simulink model "CaseStudyII_9_Bus"  (R2020a)
settings: Solver=FixedStepAuto  StartTime=0.0  StopTime=Tend  FixedStep=T_s_power  MaxStep=5.0E-5  RelTol=1e-3
values from neighbouring files (symbols this model uses):
  B_s46 = b_s46*Cb    (= 9.5071761847e-07)    [Data_CaseStudyI.m]    (also in Data_CaseStudyII.m; Data_InitialSystem.m)
  B_s54 = b_s54*Cb    (= 1.05902722057e-06)    [Data_CaseStudyI.m]    (also in Data_CaseStudyII.m; Data_InitialSystem.m)
  B_s69 = b_s69*Cb    (= 2.15415764185e-06)    [Data_CaseStudyI.m]    (also in Data_CaseStudyII.m; Data_InitialSystem.m)
  B_s75 = b_s75*Cb    (= 1.84126323577e-06)    [Data_CaseStudyI.m]    (also in Data_CaseStudyII.m; Data_InitialSystem.m)
  B_s87 = b_s87*Cb    (= 8.96562817417e-07)    [Data_CaseStudyI.m]    (also in Data_CaseStudyII.m; Data_InitialSystem.m)
  B_s98 = b_s98*Cb    (= 1.25759482443e-06)    [Data_CaseStudyI.m]    (also in Data_CaseStudyII.m; Data_InitialSystem.m)
  C_dc_DVPP_1_2 = 0.008*(n_DVPP_1_2)    (= 0.8)    [Data_CaseStudyI.m]    (also in Data_CaseStudyII.m)
  C_dc_DVPP_1_3 = 0.008*(n_DVPP_1_3)    (= 0.4)    [Data_CaseStudyI.m]    (also in Data_CaseStudyII.m)
  C_dc_DVPP_3_1 = 0.008*(n_DVPP_3_1)    (= 1.128)    [Data_CaseStudyII.m]
  C_dc_DVPP_3_2 = 0.008*(n_DVPP_3_2)    (= 0.848)    [Data_CaseStudyII.m]
  C_dc_DVPP_3_3 = 0.008*(n_DVPP_3_3)    (= 1.28)    [Data_CaseStudyII.m]
  Dp_DVPP_3_pu = 1/dp_DVPP_3    (= 33.3333333333)    [Data_CaseStudyII.m]
  Dq1_DVPP_3_pu = 100    [Data_CaseStudyII.m]
  fb = 50    [Data_CaseStudyI.m]    (also in Data_CaseStudyII.m; Data_InitialSystem.m)
  HGov_dyn = HGov_delay*H_tr_droop    [Data_CaseStudyI.m]    (also in Data_CaseStudyII.m; Data_InitialSystem.m)
  HTurb_tot = H_water_way    [Data_CaseStudyI.m]    (also in Data_CaseStudyII.m; Data_InitialSystem.m)
  I_m_DVPP_1_2 = 2/3*Sb_DVPP_1_2/V_m_DVPP_1_2    [Data_CaseStudyI.m]    (also in Data_CaseStudyII.m)
  I_m_DVPP_1_3 = 2/3*Sb_DVPP_1_3/V_m_DVPP_1_3    [Data_CaseStudyI.m]    (also in Data_CaseStudyII.m)
  I_m_DVPP_3_1 = 2/3*Sb_DVPP_3_1/V_m_DVPP_3_1    [Data_CaseStudyII.m]
  I_m_DVPP_3_2 = 2/3*Sb_DVPP_3_2/V_m_DVPP_3_2    [Data_CaseStudyII.m]
  I_m_DVPP_3_3 = 2/3*Sb_DVPP_3_3/V_m_DVPP_3_3    [Data_CaseStudyII.m]
  i_star_max = 1.3    [Data_CaseStudyI.m]    (also in Data_CaseStudyII.m)
  iabc_DVPP_1_2_0 = T0*idq0_DVPP_1_2    [Data_CaseStudyI.m]    (also in Data_CaseStudyII.m)
  iabc_DVPP_1_3_0 = T0*idq0_DVPP_1_3    [Data_CaseStudyI.m]    (also in Data_CaseStudyII.m)
  iabc_DVPP_3_1_0 = T0*idq0_DVPP_3_1    [Data_CaseStudyII.m]
  iabc_DVPP_3_2_0 = T0*idq0_DVPP_3_2    [Data_CaseStudyII.m]
  iabc_DVPP_3_3_0 = T0*idq0_DVPP_3_3    [Data_CaseStudyII.m]
  K2_DVPP_1 = [-0.0221795494247 -1.60799665656 0.160449825826 -2.94803557381 -11.8081988371 -9.75170960256 0.00463021906909 -49.1667298155]    [ControlGains_DVPP1.mat]
  K3_DVPP_1 = [-0.0591512752956 -1.61493903379 -27.2946107927 -16.2119211358 -14.3657419818 2.05688388773 -2.27328406162 0.146700393037 -150.920793597]    [ControlGains_DVPP1.mat]
  k_dc_DVPP_1_2 = eta_DVPP_1_2/(Vdc_n_DVPP_1_2*m_p_DVPP_1_2)    [Data_CaseStudyI.m]    (also in Data_CaseStudyII.m)
  k_dc_DVPP_1_3 = eta_DVPP_1_3/(Vdc_n_DVPP_1_3*m_p_DVPP_1_3)    [Data_CaseStudyI.m]    (also in Data_CaseStudyII.m)
  k_dc_DVPP_3_1 = eta_DVPP_3_1/(Vdc_n_DVPP_3_1*m_p_DVPP_3_1)    [Data_CaseStudyII.m]
  k_dc_DVPP_3_2 = eta_DVPP_3_2/(Vdc_n_DVPP_3_2*m_p_DVPP_3_2)    [Data_CaseStudyII.m]
  k_dc_DVPP_3_3 = eta_DVPP_3_3/(Vdc_n_DVPP_3_3*m_p_DVPP_3_3)    [Data_CaseStudyII.m]
  ki_i_pu = 1.19    [Data_CaseStudyI.m]    (also in Data_CaseStudyII.m)
  ki_pll = 1700    [Data_CaseStudyI.m]    (also in Data_CaseStudyII.m)
  ki_q_pu = 0.005    [Data_CaseStudyI.m]    (also in Data_CaseStudyII.m)
  kp_i_pu = 0.73    [Data_CaseStudyI.m]    (also in Data_CaseStudyII.m)
  kp_pll = 150    [Data_CaseStudyI.m]    (also in Data_CaseStudyII.m)
  kp_q_pu = 0.05    [Data_CaseStudyI.m]    (also in Data_CaseStudyII.m)
  L1_DVPP_1_2_pu = 0.0186/m_DVPP_1_2    (= 0.000372)    [Data_CaseStudyI.m]    (also in Data_CaseStudyII.m)
  L1_DVPP_1_3_pu = 0.0186/m_DVPP_1_3    (= 0.000744)    [Data_CaseStudyI.m]    (also in Data_CaseStudyII.m)
  L1_DVPP_3_1_pu = 0.0186/m_DVPP_3_1    (= 0.000263829787234)    [Data_CaseStudyII.m]
  L1_DVPP_3_2_pu = 0.0186/m_DVPP_3_2    (= 0.000350943396226)    [Data_CaseStudyII.m]
  L1_DVPP_3_3_pu = 0.0186/m_DVPP_3_3    (= 0.0002325)    [Data_CaseStudyII.m]
  l1_MVHV1 = 0    [Data_CaseStudyI.m]    (also in Data_CaseStudyII.m; Data_InitialSystem.m)
  l1_MVHV2 = 0    [Data_CaseStudyI.m]    (also in Data_CaseStudyII.m; Data_InitialSystem.m)
  l1_MVHV3 = 0    [Data_CaseStudyI.m]    (also in Data_CaseStudyII.m; Data_InitialSystem.m)
  L2_DVPP_1_2_pu = L1_DVPP_1_2_pu    (= 0.000372)    [Data_CaseStudyI.m]    (also in Data_CaseStudyII.m)
  L2_DVPP_1_3_pu = L1_DVPP_1_3_pu    (= 0.000744)    [Data_CaseStudyI.m]    (also in Data_CaseStudyII.m)
  L2_DVPP_3_1_pu = L1_DVPP_3_1_pu    (= 0.000263829787234)    [Data_CaseStudyII.m]
  L2_DVPP_3_2_pu = L1_DVPP_3_2_pu    (= 0.000350943396226)    [Data_CaseStudyII.m]
  L2_DVPP_3_3_pu = L1_DVPP_3_3_pu    (= 0.0002325)    [Data_CaseStudyII.m]
  l2_MVHV1 = l_s14    (= 0.0576)    [Data_CaseStudyI.m]    (also in Data_CaseStudyII.m; Data_InitialSystem.m)
  l2_MVHV2 = l_s72    (= 0.0625)    [Data_CaseStudyI.m]    (also in Data_CaseStudyII.m; Data_InitialSystem.m)
  l2_MVHV3 = l_s39    (= 0.0586)    [Data_CaseStudyI.m]    (also in Data_CaseStudyII.m; Data_InitialSystem.m)
  l_f_DVPP_1_2 = L_f_DVPP_1_2*w_b/Zb_DVPP_1_2    [Data_CaseStudyI.m]    (also in Data_CaseStudyII.m)
  L_f_DVPP_1_2 = (1/(n_DVPP_1_2))*600*10^-6    (= 6e-06)    [Data_CaseStudyI.m]    (also in Data_CaseStudyII.m)
  l_f_DVPP_1_3 = L_f_DVPP_1_3*w_b/Zb_DVPP_1_3    [Data_CaseStudyI.m]    (also in Data_CaseStudyII.m)
  L_f_DVPP_1_3 = (1/(n_DVPP_1_3))*600*10^-6    (= 1.2e-05)    [Data_CaseStudyI.m]    (also in Data_CaseStudyII.m)
  l_f_DVPP_3_1 = L_f_DVPP_3_1*w_b/Zb_DVPP_3_1    [Data_CaseStudyII.m]
  L_f_DVPP_3_1 = (1/(n_DVPP_3_1))*600*10^-6    (= 4.25531914894e-06)    [Data_CaseStudyII.m]
  l_f_DVPP_3_2 = L_f_DVPP_3_2*w_b/Zb_DVPP_3_2    [Data_CaseStudyII.m]
  L_f_DVPP_3_2 = (1/(n_DVPP_3_2))*600*10^-6    (= 5.66037735849e-06)    [Data_CaseStudyII.m]
  l_f_DVPP_3_3 = L_f_DVPP_3_3*w_b/Zb_DVPP_3_3    [Data_CaseStudyII.m]
  L_f_DVPP_3_3 = (1/(n_DVPP_3_3))*600*10^-6    (= 3.75e-06)    [Data_CaseStudyII.m]
  L_s46 = l_s46*Lb    (= 0.154915055408)    [Data_CaseStudyI.m]    (also in Data_CaseStudyII.m; Data_InitialSystem.m)
  L_s54 = l_s54*Lb    (= 0.143128040323)    [Data_CaseStudyI.m]    (also in Data_CaseStudyII.m; Data_InitialSystem.m)
  L_s69 = l_s69*Lb    (= 0.286256080645)    [Data_CaseStudyI.m]    (also in Data_CaseStudyII.m; Data_InitialSystem.m)
  L_s75 = l_s75*Lb    (= 0.271101346964)    [Data_CaseStudyI.m]    (also in Data_CaseStudyII.m; Data_InitialSystem.m)
  L_s87 = l_s87*Lb    (= 0.12123786945)    [Data_CaseStudyI.m]    (also in Data_CaseStudyII.m; Data_InitialSystem.m)
  L_s98 = l_s98*Lb    (= 0.16973301723)    [Data_CaseStudyI.m]    (also in Data_CaseStudyII.m; Data_InitialSystem.m)
  LPV_K1_DVPP_3 = [0.014519129833 -1.24253756746e-17 -0.00331576987938 -1.41950397655e-17 -0.00331577010739 -1.6423216922e-19 0.0145191298795 1.47256053017e-18 1.92456501739e-17 0.00968260817745 7.5102914291e-19 0.0096826081765 ... (80 elements, 8x10)]    [ControlGains_DVPP3_LPV.mat]
  LPV_K2_DVPP_3 = [0.0299413265511 -2.72480441208e-16 -0.00563144274341 -6.63344905835e-17 -0.00563144273182 -1.08918556426e-16 0.0299413268326 -1.32404731664e-16 -4.78559537004e-17 -0.00914230292149 -8.50409089014e-21 -0.00914230292147 ... (80 elements, 8x10)]    [ControlGains_DVPP3_LPV.mat]
  LPV_K3_DVPP_3 = [-0.0173301370849 5.00398589077e-17 -0.0636125194304 3.31757376688e-17 -0.0636125164794 5.41726806116e-17 -0.017330137145 2.43427565927e-17 -0.0400570975704 -5.68753124238e-17 -0.0574012283733 2.45717741258e-17 ... (192 elements, 16x12)]    [ControlGains_DVPP3_LPV.mat]
  Mp_DVPP_3_pu = 13    [Data_CaseStudyII.m]
  P_L = pL*Sb    (= 300000000)    [Data_CaseStudyI.m]    (also in Data_CaseStudyII.m; Data_InitialSystem.m)
  p_set_bus1 = P_set_bus1/SbSG1    (= 0.731707317073)    [Data_CaseStudyI.m]    (also in Data_CaseStudyII.m; Data_InitialSystem.m)
  p_set_bus2 = P_set_bus2/SbSG2    (= 0.756707317073)    [Data_CaseStudyI.m]    (also in Data_CaseStudyII.m; Data_InitialSystem.m)
  Pb_DVPP_3_1 = 37e6    (= 37000000)    [Data_CaseStudyII.m]
  Pb_DVPP_3_2 = 28e6    (= 28000000)    [Data_CaseStudyII.m]
  Pb_DVPP_3_3 = 0e6    (= 0)    [Data_CaseStudyII.m]
  pset_DVPP_1_1 = P_set_bus1/SbSG1    (= 0.731707317073)    [Data_CaseStudyI.m]    (also in Data_CaseStudyII.m)
  pset_DVPP_1_2 = 0    [Data_CaseStudyI.m]    (also in Data_CaseStudyII.m)
  pset_DVPP_1_3 = 0    [Data_CaseStudyI.m]    (also in Data_CaseStudyII.m)
  pset_DVPP_3_1 = (0.6*P_set_bus3)/Sb_DVPP_3_1    (= 0.398546964193)    [Data_CaseStudyII.m]
  pset_DVPP_3_2 = (0.4*P_set_bus3)/Sb_DVPP_3_2    (= 0.353428439945)    [Data_CaseStudyII.m]
  pset_DVPP_3_3 = 0    [Data_CaseStudyII.m]
  Q_L = qL*Sb    (= 82500000)    [Data_CaseStudyI.m]    (also in Data_CaseStudyII.m; Data_InitialSystem.m)
  qset_DVPP_1_2 = 0    [Data_CaseStudyI.m]    (also in Data_CaseStudyII.m)
  qset_DVPP_1_3 = 0    [Data_CaseStudyI.m]    (also in Data_CaseStudyII.m)
  qset_DVPP_3_1 = 0    [Data_CaseStudyII.m]
  qset_DVPP_3_2 = 0    [Data_CaseStudyII.m]
  qset_DVPP_3_3 = 0    [Data_CaseStudyII.m]
  R1_DVPP_1_2_pu = 0.00734/m_DVPP_1_2    (= 0.0001468)    [Data_CaseStudyI.m]    (also in Data_CaseStudyII.m)
  R1_DVPP_1_3_pu = 0.00734/m_DVPP_1_3    (= 0.0002936)    [Data_CaseStudyI.m]    (also in Data_CaseStudyII.m)
  R1_DVPP_3_1_pu = 0.00734/m_DVPP_3_1    (= 0.000104113475177)    [Data_CaseStudyII.m]
  R1_DVPP_3_2_pu = 0.00734/m_DVPP_3_2    (= 0.000138490566038)    [Data_CaseStudyII.m]
  R1_DVPP_3_3_pu = 0.00734/m_DVPP_3_3    (= 9.175e-05)    [Data_CaseStudyII.m]
  r1_MVHV1 = 1e-6    (= 1e-06)    [Data_CaseStudyI.m]    (also in Data_CaseStudyII.m; Data_InitialSystem.m)
  r1_MVHV2 = 1e-6    (= 1e-06)    [Data_CaseStudyI.m]    (also in Data_CaseStudyII.m; Data_InitialSystem.m)
  r1_MVHV3 = 1e-6    (= 1e-06)    [Data_CaseStudyI.m]    (also in Data_CaseStudyII.m; Data_InitialSystem.m)
  R2_DVPP_1_2_pu = R1_DVPP_1_2_pu    (= 0.0001468)    [Data_CaseStudyI.m]    (also in Data_CaseStudyII.m)
  R2_DVPP_1_3_pu = R1_DVPP_1_3_pu    (= 0.0002936)    [Data_CaseStudyI.m]    (also in Data_CaseStudyII.m)
  R2_DVPP_3_1_pu = R1_DVPP_3_1_pu    (= 0.000104113475177)    [Data_CaseStudyII.m]
  R2_DVPP_3_2_pu = R1_DVPP_3_2_pu    (= 0.000138490566038)    [Data_CaseStudyII.m]
  R2_DVPP_3_3_pu = R1_DVPP_3_3_pu    (= 9.175e-05)    [Data_CaseStudyII.m]
  r2_MVHV1 = 1e-6    (= 1e-06)    [Data_CaseStudyI.m]    (also in Data_CaseStudyII.m; Data_InitialSystem.m)
  r2_MVHV2 = 1e-6    (= 1e-06)    [Data_CaseStudyI.m]    (also in Data_CaseStudyII.m; Data_InitialSystem.m)
  r2_MVHV3 = 1e-6    (= 1e-06)    [Data_CaseStudyI.m]    (also in Data_CaseStudyII.m; Data_InitialSystem.m)
  R_dc_DVPP_1_2 = (Vdc_n_DVPP_1_2/(0.05*(Sb_DVPP_1_2)/Vdc_n_DVPP_1_2))    [Data_CaseStudyI.m]    (also in Data_CaseStudyII.m)
  R_dc_DVPP_1_3 = (Vdc_n_DVPP_1_3/(0.05*(Sb_DVPP_1_3)/Vdc_n_DVPP_1_3))    [Data_CaseStudyI.m]    (also in Data_CaseStudyII.m)
  R_dc_DVPP_3_1 = (Vdc_n_DVPP_3_1/(0.05*(Sb_DVPP_3_1)/Vdc_n_DVPP_3_1))    [Data_CaseStudyII.m]
  R_dc_DVPP_3_2 = (Vdc_n_DVPP_3_2/(0.05*(Sb_DVPP_3_2)/Vdc_n_DVPP_3_2))    [Data_CaseStudyII.m]
  R_dc_DVPP_3_3 = (Vdc_n_DVPP_3_3/(0.05*(Sb_DVPP_3_3)/Vdc_n_DVPP_3_3))    [Data_CaseStudyII.m]
  r_f_DVPP_1_2 = R_f_DVPP_1_2/Zb_DVPP_1_2    [Data_CaseStudyI.m]    (also in Data_CaseStudyII.m)
  R_f_DVPP_1_2 = 0.02/n_DVPP_1_2    (= 0.0002)    [Data_CaseStudyI.m]    (also in Data_CaseStudyII.m)
  r_f_DVPP_1_3 = R_f_DVPP_1_3/Zb_DVPP_1_3    [Data_CaseStudyI.m]    (also in Data_CaseStudyII.m)
  R_f_DVPP_1_3 = 0.02/n_DVPP_1_3    (= 0.0004)    [Data_CaseStudyI.m]    (also in Data_CaseStudyII.m)
  r_f_DVPP_3_1 = R_f_DVPP_3_1/Zb_DVPP_3_1    [Data_CaseStudyII.m]
  ... (+104 more)
undefined symbols (not defined in the file or in its folder): A, B, C, Continuous, Dd, Efd0, gcbh, i_dc, Ka, Kf, p2set, SbSM2, sps_rtmsupport, spsST1AModel, Ta, Tb, Tb1, Tc, Tc1, Tf, VA0, VAmax, VAmin, VImax, VImin, VRmax, VRmin
libraries: powerlib x95, powerlib_meascontrol x41, cstblocks x15, sps_avr x1, simulink_extras x1, simulink x1
(part 4 of 5)

== system CaseStudyII_9_Bus/STATCOM with Battery/Power Controllers1 ==
  Q_abc : Inport
  Delta x_c : Inport  Port=2
  w_pll : Inport  Port=3
  P_abc : Inport  Port=4
  P_set : Inport  Port=5
  |V| : Inport  Port=6
  Q_set : Inport  Port=7
  theta1_p : Inport  Port=8
  theta2_p : Inport  Port=9
  theta3_q : Inport  Port=10
  0 : Constant  Value=0
  DVPP State Feedback Controller : Subsystem
  Mux : Mux  Inputs=3
  i_star_dq0 : Outport
  p_des : Outport  Port=2
  q_des : Outport  Port=3
  PQ_des_DVPP3 : Outport  Port=4
  wires:
  0/1 -> Mux/3
  DVPP State Feedback Controller/1(i_star_d) -> Mux/1
  DVPP State Feedback Controller/3(p_des) -> p_des/1
  Q_abc/1 -> DVPP State Feedback Controller/5(Q_abc)
  |V|/1 -> DVPP State Feedback Controller/2("|V| ")
  DVPP State Feedback Controller/2(i_star_q) -> Mux/2
  DVPP State Feedback Controller/4(q_des) -> q_des/1
  w_pll/1 -> DVPP State Feedback Controller/1(w_pll)
  P_abc/1 -> DVPP State Feedback Controller/3(P_abc)
  P_set/1 -> DVPP State Feedback Controller/4(P_set)
  Delta x_c/1 -> DVPP State Feedback Controller/6(Delta_x_c)
  Mux/1 -> i_star_dq0/1
  Q_set/1 -> DVPP State Feedback Controller/7(Q_set)
  theta1_p/1 -> DVPP State Feedback Controller/8(theta1_p)
  theta2_p/1 -> DVPP State Feedback Controller/9(theta2_q)
  theta3_q/1 -> DVPP State Feedback Controller/10(theta3_q)
  DVPP State Feedback Controller/5(PQ_des_DVPP3) -> PQ_des_DVPP3/1

== system CaseStudyII_9_Bus/STATCOM with Battery/Reference current limitation ==
  i_star_dq0 : Inport
  i_star_max : Inport  Port=2
  Demux1 : Demux  Outputs=3
  Demux2 : Demux  Outputs=3
  Divide : Product  Inputs=*/
  Minus : Sum  Inputs=+-
  Minus1 : Sum  Inputs=+++
  Minus4 : Sum  Inputs=+++
  Product{,1..4,6..7} (7 alike) : Product  RndMeth=Zero
  Saturation1 : Saturate  UpperLimit=inf  LowerLimit=0
  Sign : Signum
  Sqrt1 : Sqrt  SaturateOnIntegerOverflow=on
  Sqrt2 : Sqrt  SaturateOnIntegerOverflow=on
  Switch1 : Switch  Threshold=1
  i_star_dq0_lim : Outport  VectorParamsAs1DForOutWhenUnconnected=off
  ||i_star_dq0|| : Outport  Port=2  VectorParamsAs1DForOutWhenUnconnected=off
  ||i_star_dq0_lim|| : Outport  Port=3  VectorParamsAs1DForOutWhenUnconnected=off
  wires:
  Sqrt2/1 -> ||i_star_dq0_lim||/1
  Minus1/1 -> Sqrt2/1
  Demux2/2 -> Product3/2, Product3/1
  Product3/1 -> Minus1/2
  Demux2/1 -> Product2/1, Product2/2
  Product4/1 -> Minus1/3
  Demux2/3 -> Product4/2, Product4/1
  Product2/1 -> Minus1/1
  i_star_max/1 -> Product6/2, Minus/2
  i_star_dq0/1 -> Switch1/3, Demux1/1, Divide/1
  Demux1/3 -> Product7/2, Product7/1
  Product7/1 -> Minus4/3
  Product6/1 -> Switch1/1
  Divide/1 -> Product6/1
  Sign/1 -> Switch1/2
  Saturation1/1 -> Sign/1
  Demux1/2 -> Product1/2, Product1/1
  Product/1 -> Minus4/1
  Product1/1 -> Minus4/2
  Demux1/1 -> Product/1, Product/2
  Minus4/1 -> Sqrt1/1
  Sqrt1/1 -> Minus/1, ||i_star_dq0||/1, Divide/2
  Minus/1 -> Saturation1/1
  Switch1/1 -> Demux2/1, i_star_dq0_lim/1

== system CaseStudyII_9_Bus/Supercapacitor/Converter State Deviation ==
  i_dq0 : Inport
  x_id : Inport  Port=2
  pset : Inport  Port=3
  Constant1 : Constant  Value=xid0_DVPP_1_3_pu
  Demux2 : Demux  Outputs=3
  Gain : Gain  Gain=1/vd0_DVPP_1_3_pu
  Mux : Mux  Inputs=2
  Sum : Sum  Inputs=-+|
  Sum1 : Sum  Inputs=|+-
  Delta x_c : Outport
  wires:
  i_dq0/1 -> Demux2/1
  pset/1 -> Gain/1
  Sum/1 -> Mux/1
  Demux2/1 -> Sum/2
  Gain/1 -> Sum/1
  x_id/1 -> Sum1/1
  Constant1/1 -> Sum1/2
  Mux/1 -> Delta x_c/1
  Sum1/1 -> Mux/2

== system CaseStudyII_9_Bus/Supercapacitor/Current Loop ==
  i_star_dq0 : Inport
  v_dq0 : Inport  Port=2
  i_dq0 : Inport  Port=3
  w_pll : Inport  Port=4
  Demux : Demux  Outputs=2
  Demux1 : Demux  Outputs=2
  Demux2 : Demux  Outputs=2
  Gain : Gain  Gain=kp_i_pu
  Gain1 : Gain  Gain=ki_i_pu
  Gain2 : Gain  Gain=kp_i_pu
  Gain3 : Gain  Gain=ki_i_pu
  Gain4 : Gain  Gain=w_b
  Integrator1 : Integrator  InitialCondition=xid0_DVPP_1_3_pu
  Integrator2 : Integrator  InitialCondition=xiq0_DVPP_1_3_pu
  Memory2 : Memory
  Mux : Mux  Inputs=3
  Product : Product
  Product1 : Product
  Rf : Gain  Gain=r_f_DVPP_1_3
  Rf1 : Gain  Gain=r_f_DVPP_1_3
  Selector1 : Selector  InputPortWidth=3  IndexOptions=Index vector (dialog)  Indices=[1 2]  OutputSizes=1
  Selector2 : Selector  InputPortWidth=3  IndexOptions=Index vector (dialog)  Indices=[1 2]  OutputSizes=1
  Selector3 : Selector  InputPortWidth=3  IndexOptions=Index vector (dialog)  Indices=[1 2]  OutputSizes=1
  Sum : Sum  Inputs=|+-
  Sum1 : Sum
  Sum2 : Sum  Inputs=|+-+
  Sum3 : Sum  Inputs=|++
  Sum4 : Sum
  Sum5 : Sum  Inputs=+++|
  Sum6 : Sum  Inputs=-+|
  Sum7 : Sum  Inputs=++|
  vs_0* : Constant  Value=0
  w*Lf : Gain  Gain=l_f_DVPP_1_3/w_b
  w*Lf1 : Gain  Gain=l_f_DVPP_1_3/w_b
  v_s_ref_dq0 : Outport  VectorParamsAs1DForOutWhenUnconnected=off
  x_id : Outport  Port=2  VectorParamsAs1DForOutWhenUnconnected=off
  wires:
  vs_0*/1 -> Mux/3
  Selector3/1 -> Demux2/1
  i_dq0/1 -> Selector2/1
  Selector2/1 -> Demux1/1
  Mux/1 -> v_s_ref_dq0/1
  Sum2/1 -> Sum3/1
  v_dq0/1 -> Selector3/1
  i_star_dq0/1 -> Selector1/1
  w*Lf/1 -> Sum2/2
  Sum7/1 -> Mux/2  "vs_q*"
  Sum3/1 -> Mux/1  "vs_d*"
  Sum5/1 -> Sum7/2
  Rf/1 -> Sum2/3
  Rf1/1 -> Sum5/3
  Sum/1 -> Integrator1/1, Gain/1
  Sum1/1 -> Sum2/1
  Selector1/1 -> Demux/1
  Demux/2 -> Sum6/2
  Demux/1 -> Sum/1
  w*Lf1/1 -> Sum5/1
  Demux2/1 -> Sum3/2
  Demux2/2 -> Sum7/1
  Demux1/1 -> Product/1, Rf/1, Sum/2
  Demux1/2 -> Product1/1, Rf1/1, Sum6/1
  Gain/1 -> Sum1/1
  Gain1/1 -> Sum1/2
  Gain2/1 -> Sum4/1
  Sum6/1 -> Integrator2/1, Gain2/1
  Sum4/1 -> Sum5/2
  Gain3/1 -> Sum4/2
  Integrator2/1 -> Gain3/1
  Integrator1/1 -> Memory2/1, Gain1/1
  w_pll/1 -> Gain4/1
  Product/1 -> w*Lf1/1
  Product1/1 -> w*Lf/1
  Gain4/1 -> Product1/2, Product/2
  Memory2/1 -> x_id/1

== system CaseStudyII_9_Bus/Supercapacitor/PLL ==
  v_abc : Inport
  Display : Display
  Gain : Gain  Gain=1/fb
  Integrator3 : Integrator  InitialCondition=xpll0_pu
  Selector : Selector  InputPortWidth=3  IndexOptions=Index vector (dialog)  Indices=2  OutputSizes=1
  Subsystem : Subsystem
  abc to dq0 : powerlib_meascontrol/Transformations/abc to dq0  Alignment=90 degrees behind phase A axis
  theta_pll : Outport  VectorParamsAs1DForOutWhenUnconnected=off
  v_dq0 : Outport  Port=2  VectorParamsAs1DForOutWhenUnconnected=off
  w_pll : Outport  Port=3  VectorParamsAs1DForOutWhenUnconnected=off
  x_pll : Outport  Port=4  VectorParamsAs1DForOutWhenUnconnected=off
  wires:
  Gain/1 -> w_pll/1
  Integrator3/1 -> x_pll/1
  v_abc/1 -> Subsystem/1(Vabc), abc to dq0/1
  abc to dq0/1 -> Selector/1, v_dq0/1
  Subsystem/1(Freq) -> Display/1, Gain/1
  Subsystem/2(wt) -> abc to dq0/2, theta_pll/1
  Selector/1 -> Integrator3/1

== system CaseStudyII_9_Bus/Supercapacitor/Power Controllers ==
  Q_abc : Inport
  w_pll : Inport  Port=2
  P_abc : Inport  Port=3
  Q_set : Inport  Port=4
  Delta x_c : Inport  Port=5
  P_set : Inport  Port=6
  0 : Constant  Value=0
  DVPP State Feedback Controller for Active Power Control : Subsystem
  Mux : Mux  Inputs=3
  Reactive Power Controller PI-droop control : Subsystem
  i_star_dq0 : Outport
  p_des : Outport  Port=2
  wires:
  Mux/1 -> i_star_dq0/1
  0/1 -> Mux/3
  DVPP State Feedback Controller for Active Power Control/2(i_star_d) -> Mux/1
  DVPP State Feedback Controller for Active Power Control/1(p_des) -> p_des/1
  w_pll/1 -> DVPP State Feedback Controller for Active Power Control/1(w_pll)
  P_abc/1 -> DVPP State Feedback Controller for Active Power Control/2(P_abc)
  Reactive Power Controller PI-droop control/1(i_star_q) -> Mux/2
  Q_abc/1 -> Reactive Power Controller PI-droop control/1(Q_abc)
  Q_set/1 -> Reactive Power Controller PI-droop control/2(Qset)
  Delta x_c/1 -> DVPP State Feedback Controller for Active Power Control/3(Delta_x_c)
  P_set/1 -> DVPP State Feedback Controller for Active Power Control/4(P_set)

== system CaseStudyII_9_Bus/Supercapacitor/Reference current limitation ==
  i_star_dq0 : Inport
  i_star_max : Inport  Port=2
  Demux1 : Demux  Outputs=3
  Demux2 : Demux  Outputs=3
  Divide : Product  Inputs=*/
  Minus : Sum  Inputs=+-
  Minus1 : Sum  Inputs=+++
  Minus4 : Sum  Inputs=+++
  Product{,1..4,6..7} (7 alike) : Product  RndMeth=Zero
  Saturation1 : Saturate  UpperLimit=inf  LowerLimit=0
  Sign : Signum
  Sqrt1 : Sqrt  SaturateOnIntegerOverflow=on
  Sqrt2 : Sqrt  SaturateOnIntegerOverflow=on
  Switch1 : Switch  Threshold=1
  i_star_dq0_lim : Outport  VectorParamsAs1DForOutWhenUnconnected=off
  ||i_star_dq0|| : Outport  Port=2  VectorParamsAs1DForOutWhenUnconnected=off
  ||i_star_dq0_lim|| : Outport  Port=3  VectorParamsAs1DForOutWhenUnconnected=off
  wires:
  Sqrt2/1 -> ||i_star_dq0_lim||/1
  Minus1/1 -> Sqrt2/1
  Demux2/2 -> Product3/2, Product3/1
  Product3/1 -> Minus1/2
  Demux2/1 -> Product2/1, Product2/2
  Product4/1 -> Minus1/3
  Demux2/3 -> Product4/2, Product4/1
  Product2/1 -> Minus1/1
  i_star_max/1 -> Product6/2, Minus/2
  i_star_dq0/1 -> Switch1/3, Demux1/1, Divide/1
  Switch1/1 -> i_star_dq0_lim/1, Demux2/1
  Demux1/3 -> Product7/2, Product7/1
  Product7/1 -> Minus4/3
  Product6/1 -> Switch1/1
  Divide/1 -> Product6/1
  Sign/1 -> Switch1/2
  Saturation1/1 -> Sign/1
  Demux1/2 -> Product1/2, Product1/1
  Product/1 -> Minus4/1
  Product1/1 -> Minus4/2
  Demux1/1 -> Product/1, Product/2
  Minus4/1 -> Sqrt1/1
  Sqrt1/1 -> Minus/1, ||i_star_dq0||/1, Divide/2
  Minus/1 -> Saturation1/1

== system CaseStudyII_9_Bus/Synchronous Generator 1 Hydro Turbine/Govenor ==
  speed_ref : Inport
  speed : Inport  Port=2
  P_set : Inport  Port=3
  1/droop : Gain  Gain=(-1/Rg)
  Delta speed : Sum  Inputs=-+|
  Govenor Dynamics : cstblocks/LTI System  sys=ss(HGov_dyn)  IC=[1 1.0617]
  Sum : Sum  Inputs=++|
  throttle : Outport  VectorParamsAs1DForOutWhenUnconnected=off
  wires:
  speed/1 -> Delta speed/2
  speed_ref/1 -> Delta speed/1
  Govenor Dynamics/1 -> throttle/1
  Delta speed/1 -> 1/droop/1
  Sum/1 -> Govenor Dynamics/1
  1/droop/1 -> Sum/2  "Pm"
  P_set/1 -> Sum/1

== system CaseStudyII_9_Bus/Synchronous Machine 2 reheat steam turbine/Govenor ==
  speed_ref : Inport
  speed : Inport  Port=2
  P_set : Inport  Port=3
  1/droop : Gain  Gain=(-1/Rg)
  Delta speed : Sum  Inputs=-+|
  Govenor Dynamics : cstblocks/LTI System  sys=ss(SGov_dyn)  IC=[p_set_bus2/2.5]
  Sum : Sum  Inputs=++|
  throttle : Outport  VectorParamsAs1DForOutWhenUnconnected=off
  wires:
  speed/1 -> Delta speed/2
  speed_ref/1 -> Delta speed/1
  Govenor Dynamics/1 -> throttle/1
  Delta speed/1 -> 1/droop/1
  1/droop/1 -> Sum/2  "Pm"
  Sum/1 -> Govenor Dynamics/1
  P_set/1 -> Sum/1

== system CaseStudyII_9_Bus/Synchronous Machine 2 reheat steam turbine/ST1A Excitation System ==
  Vref : Inport
  Vt : Inport  Port=2
  Ifd : Inport  Port=3
  Vstab : Inport  Port=4
  Model : Subsystem  AncestorBlock=spsST1AModel/Continuous  mask(Excitation System){}
  Efd : Outport  VectorParamsAs1DForOutWhenUnconnected=off
  wires:
  Vstab/1 -> Model/4(Vstab)
  Ifd/1 -> Model/3(Ifd)
  Vref/1 -> Model/1(Vref)
  Vt/1 -> Model/2(Vt)
  Model/1(Efd) -> Efd/1

== system CaseStudyII_9_Bus/Wind /Converter State Deviation for DVPP with DC side1 ==
  i_dq0 : Inport
  Pset : Inport  Port=2
  Qset : Inport  Port=3
  x_id : Inport  Port=4
  x_iq : Inport  Port=5
  Demux2 : Demux  Outputs=3
  Gain : Gain  Gain=1/vd0_DVPP_3_1_pu
  Gain1 : Gain  Gain=-1/vd0_DVPP_3_1_pu
  Mux : Mux
  Sum1 : Sum  Inputs=+-
  Sum2 : Sum  Inputs=-+
  Sum3 : Sum  Inputs=+-
  Sum4 : Sum  Inputs=+-
  x_id_1_pu : Constant  Value=xid0_DVPP_3_1_pu
  x_iq_1_pu : Constant  Value=xiq0_DVPP_3_1_pu
  Delta x_c : Outport
  wires:
  i_dq0/1 -> Demux2/1
  Demux2/1 -> Sum2/2
  Demux2/2 -> Sum1/1
  Sum2/1 -> Mux/1
  Sum1/1 -> Mux/2
  Gain1/1 -> Sum1/2
  Pset/1 -> Gain/1
  Gain/1 -> Sum2/1
  Qset/1 -> Gain1/1
  x_id/1 -> Sum3/1
  Sum3/1 -> Mux/3
  x_id_1_pu/1 -> Sum3/2
  Mux/1 -> Delta x_c/1
  Sum4/1 -> Mux/4
  x_iq_1_pu/1 -> Sum4/2
  x_iq/1 -> Sum4/1

== system CaseStudyII_9_Bus/Wind /Current Loop ==
  i_star_dq0 : Inport
  v_dq0 : Inport  Port=2
  i_dq0 : Inport  Port=3
  w_pll : Inport  Port=4
  Demux : Demux  Outputs=2
  Demux1 : Demux  Outputs=2
  Demux2 : Demux  Outputs=2
  Gain : Gain  Gain=kp_i_pu
  Gain1 : Gain  Gain=ki_i_pu
  Gain2 : Gain  Gain=kp_i_pu
  Gain3 : Gain  Gain=ki_i_pu
  Gain4 : Gain  Gain=w_b
  Integrator1 : Integrator  InitialCondition=xid0_DVPP_3_1_pu
  Integrator2 : Integrator  InitialCondition=xiq0_DVPP_3_1_pu
  Memory1 : Memory
  Memory2 : Memory
  Mux : Mux  Inputs=3
  Product : Product
  Product1 : Product
  Rf : Gain  Gain=r_f_DVPP_3_1
  Rf1 : Gain  Gain=r_f_DVPP_3_1
  Selector1 : Selector  InputPortWidth=3  IndexOptions=Index vector (dialog)  Indices=[1 2]  OutputSizes=1
  Selector2 : Selector  InputPortWidth=3  IndexOptions=Index vector (dialog)  Indices=[1 2]  OutputSizes=1
  Selector3 : Selector  InputPortWidth=3  IndexOptions=Index vector (dialog)  Indices=[1 2]  OutputSizes=1
  Sum : Sum  Inputs=|+-
  Sum1 : Sum
  Sum2 : Sum  Inputs=|+-+
  Sum3 : Sum  Inputs=|++
  Sum4 : Sum
  Sum5 : Sum  Inputs=+++|
  Sum6 : Sum  Inputs=-+|
  Sum7 : Sum  Inputs=++|
  vs_0* : Constant  Value=0
  w*Lf : Gain  Gain=l_f_DVPP_3_1/w_b
  w*Lf1 : Gain  Gain=l_f_DVPP_3_1/w_b
  v_s_ref_dq0 : Outport  VectorParamsAs1DForOutWhenUnconnected=off
  x_id : Outport  Port=2  VectorParamsAs1DForOutWhenUnconnected=off
  x_iq : Outport  Port=3  VectorParamsAs1DForOutWhenUnconnected=off
  wires:
  vs_0*/1 -> Mux/3
  Selector3/1 -> Demux2/1
  i_dq0/1 -> Selector2/1
  Selector2/1 -> Demux1/1
  Mux/1 -> v_s_ref_dq0/1
  Sum2/1 -> Sum3/1
  v_dq0/1 -> Selector3/1
  i_star_dq0/1 -> Selector1/1
  w*Lf/1 -> Sum2/2
  Sum7/1 -> Mux/2  "vs_q*"
  Sum3/1 -> Mux/1  "vs_d*"
  Sum5/1 -> Sum7/2
  Rf/1 -> Sum2/3
  Rf1/1 -> Sum5/3
  Sum/1 -> Integrator1/1, Gain/1
  Sum1/1 -> Sum2/1
  Selector1/1 -> Demux/1
  Demux/2 -> Sum6/2
  Demux/1 -> Sum/1
  w*Lf1/1 -> Sum5/1
  Demux2/1 -> Sum3/2
  Demux2/2 -> Sum7/1
  Demux1/1 -> Product/1, Rf/1, Sum/2
  Demux1/2 -> Product1/1, Rf1/1, Sum6/1
  Gain/1 -> Sum1/1
  Gain1/1 -> Sum1/2
  Gain2/1 -> Sum4/1
  Sum6/1 -> Integrator2/1, Gain2/1
  Sum4/1 -> Sum5/2
  Gain3/1 -> Sum4/2
  Integrator2/1 -> Memory1/1, Gain3/1
  Integrator1/1 -> Memory2/1, Gain1/1
  w_pll/1 -> Gain4/1
  Product/1 -> w*Lf1/1
  Product1/1 -> w*Lf/1
  Gain4/1 -> Product1/2, Product/2
  Memory2/1 -> x_id/1
  Memory1/1 -> x_iq/1

== system CaseStudyII_9_Bus/Wind /PLL ==
  v_abc : Inport
  Display : Display
  Gain : Gain  Gain=1/fb
  Integrator3 : Integrator  InitialCondition=xpll0_pu
  Selector : Selector  InputPortWidth=3  IndexOptions=Index vector (dialog)  Indices=2  OutputSizes=1
  Subsystem : Subsystem
  abc to dq0 : powerlib_meascontrol/Transformations/abc to dq0  Alignment=90 degrees behind phase A axis
  theta_pll : Outport  VectorParamsAs1DForOutWhenUnconnected=off
  v_dq0 : Outport  Port=2  VectorParamsAs1DForOutWhenUnconnected=off
  w_pll : Outport  Port=3  VectorParamsAs1DForOutWhenUnconnected=off
  x_pll : Outport  Port=4  VectorParamsAs1DForOutWhenUnconnected=off
  wires:
  Gain/1 -> w_pll/1
  Integrator3/1 -> x_pll/1
  v_abc/1 -> Subsystem/1(Vabc), abc to dq0/1
  abc to dq0/1 -> Selector/1, v_dq0/1
  Subsystem/1(Freq) -> Display/1, Gain/1
  Subsystem/2(wt) -> abc to dq0/2, theta_pll/1
  Selector/1 -> Integrator3/1

== system CaseStudyII_9_Bus/Wind /Power Controllers1 ==
  Q_abc : Inport
  Delta x_c : Inport  Port=2
  w_pll : Inport  Port=3
  P_abc : Inport  Port=4
  P_set : Inport  Port=5
  |V| : Inport  Port=6
  Q_set : Inport  Port=7
  theta1_p : Inport  Port=8
  theta1_q : Inport  Port=9
  0 : Constant  Value=0
  DVPP State Feedback Controller : Subsystem
  Mux : Mux  Inputs=3
  i_star_dq0 : Outport
  p_des : Outport  Port=2
  q_des : Outport  Port=3
  wires:
  0/1 -> Mux/3
  DVPP State Feedback Controller/1(i_star_d) -> Mux/1
  DVPP State Feedback Controller/3(p_des) -> p_des/1
  Q_abc/1 -> DVPP State Feedback Controller/5(Q_abc)
  |V|/1 -> DVPP State Feedback Controller/2("|V| ")
  DVPP State Feedback Controller/2(i_star_q) -> Mux/2
  DVPP State Feedback Controller/4(q_des) -> q_des/1
  w_pll/1 -> DVPP State Feedback Controller/1(w_pll)
  P_abc/1 -> DVPP State Feedback Controller/3(P_abc)
  P_set/1 -> DVPP State Feedback Controller/4(P_set)
  Delta x_c/1 -> DVPP State Feedback Controller/6(Delta_x_c)
  Mux/1 -> i_star_dq0/1
  Q_set/1 -> DVPP State Feedback Controller/7(Q_set)
  theta1_q/1 -> DVPP State Feedback Controller/9(theta1_q)
  theta1_p/1 -> DVPP State Feedback Controller/8(theta1_p)

== system CaseStudyII_9_Bus/Wind /Reference current limitation ==
  i_star_dq0 : Inport
  i_star_max : Inport  Port=2
  Demux1 : Demux  Outputs=3
  Demux2 : Demux  Outputs=3
  Divide : Product  Inputs=*/
  Minus : Sum  Inputs=+-
  Minus1 : Sum  Inputs=+++
  Minus4 : Sum  Inputs=+++
  Product{,1..4,6..7} (7 alike) : Product  RndMeth=Zero
  Saturation1 : Saturate  UpperLimit=inf  LowerLimit=0
  Sign : Signum
  Sqrt1 : Sqrt  SaturateOnIntegerOverflow=on
  Sqrt2 : Sqrt  SaturateOnIntegerOverflow=on
  Switch1 : Switch  Threshold=1
  i_star_dq0_lim : Outport  VectorParamsAs1DForOutWhenUnconnected=off
  ||i_star_dq0|| : Outport  Port=2  VectorParamsAs1DForOutWhenUnconnected=off
  ||i_star_dq0_lim|| : Outport  Port=3  VectorParamsAs1DForOutWhenUnconnected=off
  wires:
  Sqrt2/1 -> ||i_star_dq0_lim||/1
  Minus1/1 -> Sqrt2/1
  Demux2/2 -> Product3/2, Product3/1
  Product3/1 -> Minus1/2
  Demux2/1 -> Product2/1, Product2/2
  Product4/1 -> Minus1/3
  Demux2/3 -> Product4/2, Product4/1
  Product2/1 -> Minus1/1
  i_star_max/1 -> Product6/2, Minus/2
  i_star_dq0/1 -> Switch1/3, Demux1/1, Divide/1
  Demux1/3 -> Product7/2, Product7/1
  Product7/1 -> Minus4/3
  Product6/1 -> Switch1/1
  Divide/1 -> Product6/1
  Sign/1 -> Switch1/2
  Saturation1/1 -> Sign/1
  Demux1/2 -> Product1/2, Product1/1
  Product/1 -> Minus4/1
  Product1/1 -> Minus4/2
  Demux1/1 -> Product/1, Product/2
  Minus4/1 -> Sqrt1/1
  Sqrt1/1 -> Minus/1, ||i_star_dq0||/1, Divide/2
  Minus/1 -> Saturation1/1
  Switch1/1 -> Demux2/1, i_star_dq0_lim/1

== system CaseStudyII_9_Bus/BESS/PLL/Subsystem ==
  Vabc : Inport  PortDimensions=3
  Constant : Constant  Value=2*pi*50
  Demux2 : Demux  Outputs=3
  Divide : Product  Inputs=/*
  First-Order Filter : powerlib_meascontrol/Filters/First-Order Filter  FilterType=Lowpass  Tc=0.081  Ts=0  Initialize=on  Vac_Init=[0, 0, fb]  Vdc_Init=0  PlotResponse=off  FreqRange="[0,  200,  1]"
  Gain : Gain  Gain=kp_pll
  Gain1 : Gain  Gain=ki_pll
  Gain10 : Gain  Gain=1/2/pi  SaturateOnIntegerOverflow=on  OutDataTypeStr=Inherit: Same as input  ParamDataTypeStr=Inherit: Same as input
  Integrator : Integrator
  Integrator1 : Integrator  InitialCondition=xpll0_pu
  Memory : Memory  InitialCondition=fb
  Selector : Selector  InputPortWidth=3  IndexOptions=Index vector (dialog)  Indices=2  OutputSizes=1
  Sqrt2 : Sqrt  SaturateOnIntegerOverflow=on
  Sum : Sum
  Sum1 : Sum  Inputs=++|
  Sum2 : Sum  Inputs=+++  InputSameDT=on  SaturateOnIntegerOverflow=on  OutDataTypeStr=Inherit: Same as first input
  abc to dq0 : powerlib_meascontrol/Transformations/abc to dq0  Alignment=90 degrees behind phase A axis
      settings: SourceProductBaseCode=MT,PS
  d²2 : Product  InputSameDT=on  RndMeth=Zero  SaturateOnIntegerOverflow=on  OutDataTypeStr=Inherit: Same as first input
  q²4 : Product  InputSameDT=on  RndMeth=Zero  SaturateOnIntegerOverflow=on  OutDataTypeStr=Inherit: Same as first input
  q²5 : Product  InputSameDT=on  RndMeth=Zero  SaturateOnIntegerOverflow=on  OutDataTypeStr=Inherit: Same as first input
  Freq : Outport  VectorParamsAs1DForOutWhenUnconnected=off
  wt : Outport  Port=2  VectorParamsAs1DForOutWhenUnconnected=off
  wires:
  Vabc/1 -> abc to dq0/1
  Integrator/1 -> wt/1, abc to dq0/2
  Memory/1 -> Freq/1
  Gain/1 -> Sum/1
  Gain1/1 -> Sum/2
  Integrator1/1 -> Gain1/1
  Demux2/1 -> d²2/1, d²2/2  "d"
  d²2/1 -> Sum2/1
  Demux2/3 -> q²5/1, q²5/2  "0"
  Demux2/2 -> q²4/1, q²4/2  "q"
  Sqrt2/1 -> Divide/1
  Sum2/1 -> Sqrt2/1
  q²5/1 -> Sum2/3
  abc to dq0/1 -> Demux2/1, Selector/1
  q²4/1 -> Sum2/2
  Selector/1 -> Divide/2  "Vq"
  Divide/1 -> Integrator1/1, Gain/1
  Gain10/1 -> First-Order Filter/1
  First-Order Filter/1 -> Memory/1
  Sum/1 -> Sum1/2  "W"
  Sum1/1 -> Integrator/1, Gain10/1  "W"
  Constant/1 -> Sum1/1

== system CaseStudyII_9_Bus/BESS/Power Controllers/DVPP State Feedback Controller for Active Power Control ==
  P_abc : Inport
  Delta_x_c : Inport  Port=2
  w_pll : Inport  Port=3
  Pset : Inport  Port=4
  Constant : Constant  Value=ReferenceSS2_DVPP_1.A  VectorParams1D=off
  Constant1 : Constant  Value=ReferenceSS2_DVPP_1.B  VectorParams1D=off
  Constant2 : Constant  Value=ReferenceSS2_DVPP_1.C  VectorParams1D=off
  Constant3 : Constant  Value=ReferenceSS2_DVPP_1.D  VectorParams1D=off
  Gain : Gain  Gain=K2_DVPP_1  Multiplication=Matrix(K*u)
  Gain1 : Gain  Gain=1/vd0_DVPP_1_2_pu
  Integrator : Integrator
  Mux : Mux  Inputs=3
  Scope : Scope
  Sum : Sum  Inputs=+-
  Sum1 : Sum  Inputs=++|
  Sum2 : Sum
  Sum3 : Sum  Inputs=-+
  Varying State Space : cstblocks/Linear Parameter Varying/Varying State Space  x0=0  xNames=''  OutputX=on  OutputDX=on
  w* [SI] : Constant
  p_des : Outport
  i_star_d : Outport  Port=2
  wires:
  Mux/1 -> Gain/1
  Varying State Space/1 -> Scope/1, Sum1/2
  Sum3/1 -> Integrator/1
  w* [SI]/1 -> Sum/2
  P_abc/1 -> Sum3/2
  Integrator/1 -> Mux/3
  Varying State Space/2 -> Mux/2
  Delta_x_c/1 -> Mux/1
  w_pll/1 -> Sum/1
  Constant/1 -> Varying State Space/2
  Constant1/1 -> Varying State Space/3
  Constant2/1 -> Varying State Space/4
  Constant3/1 -> Varying State Space/5
  Sum/1 -> Varying State Space/1
  Pset/1 -> Gain1/1, Sum1/1
  Sum1/1 -> Sum3/1, p_des/1
  Sum2/1 -> i_star_d/1
  Gain/1 -> Sum2/1
  Gain1/1 -> Sum2/2

== system CaseStudyII_9_Bus/BESS/Power Controllers/Reactive Power Controller PI-droop control ==
  Q_abc : Inport
  Qset : Inport  Port=2
  Gain : Gain  Gain=kp_q_pu
  Gain1 : Gain  Gain=ki_q_pu
  Integrator1 : Integrator  InitialCondition=xq0_DVPP_1_2_pu
  Sum : Sum  Inputs=-+
  Sum1 : Sum
  i_star_q : Outport
  wires:
  Q_abc/1 -> Sum/2
  Qset/1 -> Sum/1
  Sum/1 -> Integrator1/1, Gain/1
  Gain/1 -> Sum1/1
  Gain1/1 -> Sum1/2
  Integrator1/1 -> Gain1/1
  Sum1/1 -> i_star_q/1

== system CaseStudyII_9_Bus/PV/PLL/Subsystem ==
  Vabc : Inport  PortDimensions=3
  Constant : Constant  Value=2*pi*50
  Demux2 : Demux  Outputs=3
  Divide : Product  Inputs=/*
  First-Order Filter : powerlib_meascontrol/Filters/First-Order Filter  FilterType=Lowpass  Tc=0.081  Ts=0  Initialize=on  Vac_Init=[0, 0, fb]  Vdc_Init=0  PlotResponse=off  FreqRange="[0,  200,  1]"
  Gain : Gain  Gain=kp_pll
  Gain1 : Gain  Gain=ki_pll
  Gain10 : Gain  Gain=1/2/pi  SaturateOnIntegerOverflow=on  OutDataTypeStr=Inherit: Same as input  ParamDataTypeStr=Inherit: Same as input
  Integrator : Integrator
  Integrator1 : Integrator  InitialCondition=xpll0_pu
  Memory : Memory  InitialCondition=fb
  Selector : Selector  InputPortWidth=3  IndexOptions=Index vector (dialog)  Indices=2  OutputSizes=1
  Sqrt2 : Sqrt  SaturateOnIntegerOverflow=on
  Sum : Sum
  Sum1 : Sum  Inputs=++|
  Sum2 : Sum  Inputs=+++  InputSameDT=on  SaturateOnIntegerOverflow=on  OutDataTypeStr=Inherit: Same as first input
  abc to dq0 : powerlib_meascontrol/Transformations/abc to dq0  Alignment=90 degrees behind phase A axis
      settings: SourceProductBaseCode=MT,PS
  d²2 : Product  InputSameDT=on  RndMeth=Zero  SaturateOnIntegerOverflow=on  OutDataTypeStr=Inherit: Same as first input
  q²4 : Product  InputSameDT=on  RndMeth=Zero  SaturateOnIntegerOverflow=on  OutDataTypeStr=Inherit: Same as first input
  q²5 : Product  InputSameDT=on  RndMeth=Zero  SaturateOnIntegerOverflow=on  OutDataTypeStr=Inherit: Same as first input
  Freq : Outport  VectorParamsAs1DForOutWhenUnconnected=off
  wt : Outport  Port=2  VectorParamsAs1DForOutWhenUnconnected=off
  wires:
  Vabc/1 -> abc to dq0/1
  Integrator/1 -> wt/1, abc to dq0/2
  Memory/1 -> Freq/1
  Gain/1 -> Sum/1
  Gain1/1 -> Sum/2
  Integrator1/1 -> Gain1/1
  Demux2/1 -> d²2/1, d²2/2  "d"
  d²2/1 -> Sum2/1
  Demux2/3 -> q²5/1, q²5/2  "0"
  Demux2/2 -> q²4/1, q²4/2  "q"
  Sqrt2/1 -> Divide/1
  Sum2/1 -> Sqrt2/1
  q²5/1 -> Sum2/3
  abc to dq0/1 -> Demux2/1, Selector/1
  q²4/1 -> Sum2/2
  Selector/1 -> Divide/2  "Vq"
  Divide/1 -> Integrator1/1, Gain/1
  Gain10/1 -> First-Order Filter/1
  First-Order Filter/1 -> Memory/1
  Constant/1 -> Sum1/1
  Sum/1 -> Sum1/2  "W"
  Sum1/1 -> Integrator/1, Gain10/1  "W"

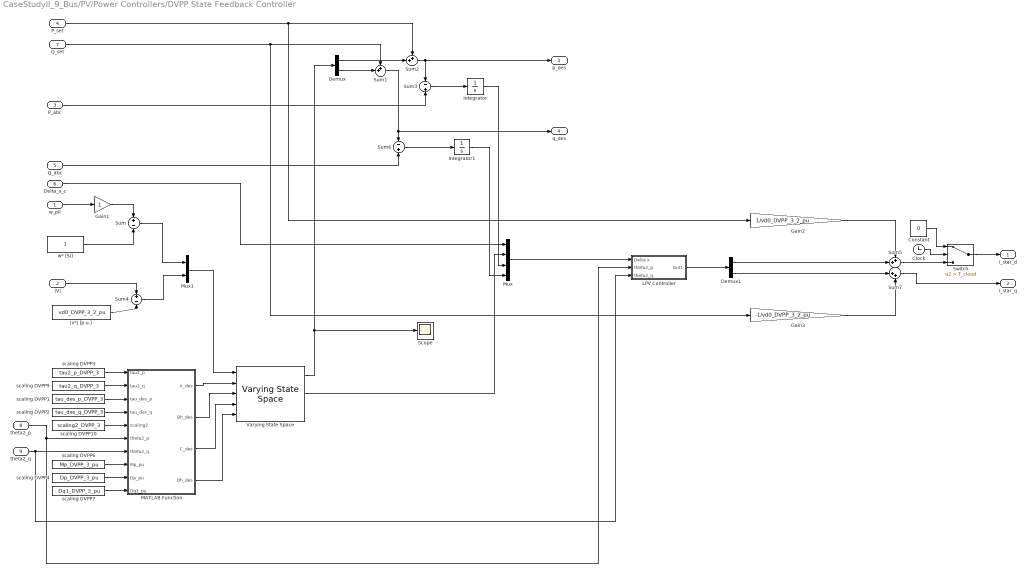
== system CaseStudyII_9_Bus/PV/Power Controllers/DVPP State Feedback Controller ==
  w_pll : Inport
  "|V| " : Inport  Port=2
  P_abc : Inport  Port=3
  P_set : Inport  Port=4
  Q_abc : Inport  Port=5
  Delta_x_c : Inport  Port=6
  Q_set : Inport  Port=7
  theta2_p : Inport  Port=8
  theta2_q : Inport  Port=9
  Clock : Clock
  Constant : Constant  Value=0
  Demux : Demux  Outputs=2
  Demux1 : Demux  Outputs=2
  Gain1 : Gain
  Gain2 : Gain  Gain=1/vd0_DVPP_3_2_pu
  Gain3 : Gain  Gain=-1/vd0_DVPP_3_2_pu
  Integrator : Integrator
  Integrator1 : Integrator
  LPV Controller : Subsystem
  MATLAB Function : MATLAB Function  TreatAsAtomicUnit=on
  Mux : Mux
  Mux1 : Mux  Inputs=2
  Scope : Scope
  Sum : Sum  Inputs=+-
  Sum1 : Sum  Inputs=++|
  Sum2 : Sum  Inputs=++|
  Sum3 : Sum  Inputs=-+
  Sum4 : Sum  Inputs=+-
  Sum5 : Sum  Inputs=++|
  Sum6 : Sum  Inputs=-+
  Sum7 : Sum  Inputs=|++
  Switch : Switch  Criteria=u2 > Threshold  Threshold=T_cloud
  Varying State Space : cstblocks/Linear Parameter Varying/Varying State Space  x0=0  xNames=''  OutputX=on  OutputDX=on
  scaling DVPP1 : Constant  Value=tau_des_p_DVPP_3
  scaling DVPP10 : Constant  Value=scaling2_DVPP_3
  scaling DVPP2 : Constant  Value=tau_des_q_DVPP_3
  scaling DVPP3 : Constant  Value=tau2_p_DVPP_3
  scaling DVPP4 : Constant  Value=Dp_DVPP_3_pu
  scaling DVPP6 : Constant  Value=Mp_DVPP_3_pu
  scaling DVPP7 : Constant  Value=Dq1_DVPP_3_pu
  scaling DVPP9 : Constant  Value=tau2_q_DVPP_3
  w* [SI] : Constant
  |v*| [p.u.] : Constant  Value=vd0_DVPP_3_2_pu
  i_star_d : Outport
  i_star_q : Outport  Port=2
  p_des : Outport  Port=3
  q_des : Outport  Port=4
  wires:
  Mux/1 -> LPV Controller/1(Delta x)
  Sum3/1 -> Integrator/1
  "|V| "/1 -> Sum4/1
  |v*| [p.u.]/1 -> Sum4/2
  w_pll/1 -> Gain1/1
  w* [SI]/1 -> Sum/2
  Sum/1 -> Mux1/1
  Mux1/1 -> Varying State Space/1
  Varying State Space/1 -> Demux/1, Scope/1
  P_abc/1 -> Sum3/2
  Q_abc/1 -> Sum6/2
  Sum6/1 -> Integrator1/1
  Integrator/1 -> Mux/3
  Integrator1/1 -> Mux/4
  Varying State Space/2 -> Mux/2
  Delta_x_c/1 -> Mux/1
  LPV Controller/1(Out1) -> Demux1/1
  Gain1/1 -> Sum/1
  Sum4/1 -> Mux1/2
  Demux/2 -> Sum1/2
  Q_set/1 -> Gain3/1, Sum1/1
  Sum1/1 -> q_des/1, Sum6/1
  Sum2/1 -> Sum3/1, p_des/1
  Demux/1 -> Sum2/2
  P_set/1 -> Gain2/1, Sum2/1
  Gain2/1 -> Sum5/1
  Demux1/1 -> Sum5/2
  Sum7/1 -> i_star_q/1
  Demux1/2 -> Sum7/1
  Gain3/1 -> Sum7/2
  scaling DVPP10/1 -> MATLAB Function/5(scaling2)
  theta2_q/1 -> LPV Controller/3(theta2_q), MATLAB Function/7(theta2_q)
  scaling DVPP6/1 -> MATLAB Function/8(Mp_pu)
  scaling DVPP4/1 -> MATLAB Function/9(Dp_pu)
  scaling DVPP3/1 -> MATLAB Function/1(tau2_p)
  scaling DVPP2/1 -> MATLAB Function/4(tau_des_q)
  scaling DVPP1/1 -> MATLAB Function/3(tau_des_p)
  scaling DVPP9/1 -> MATLAB Function/2(tau2_q)
  scaling DVPP7/1 -> MATLAB Function/10(Dq1_pu)
  MATLAB Function/1(A_des) -> Varying State Space/2
  MATLAB Function/2(Bh_des) -> Varying State Space/3
  MATLAB Function/3(C_des) -> Varying State Space/4
  MATLAB Function/4(Dh_des) -> Varying State Space/5
  theta2_p/1 -> MATLAB Function/6(theta2_p), LPV Controller/2(theta2_p)
  Switch/1 -> i_star_d/1
  Sum5/1 -> Switch/3
  Clock/1 -> Switch/2
  Constant/1 -> Switch/1

== system CaseStudyII_9_Bus/STATCOM with Battery/PLL/Subsystem ==
  Vabc : Inport  PortDimensions=3
  Constant : Constant  Value=2*pi*50
  Demux2 : Demux  Outputs=3
  Divide : Product  Inputs=/*
  First-Order Filter : powerlib_meascontrol/Filters/First-Order Filter  FilterType=Lowpass  Tc=0.081  Ts=0  Initialize=on  Vac_Init=[0, 0, fb]  Vdc_Init=0  PlotResponse=off  FreqRange="[0,  200,  1]"
  Gain : Gain  Gain=kp_pll
  Gain1 : Gain  Gain=ki_pll
  Gain10 : Gain  Gain=1/2/pi  SaturateOnIntegerOverflow=on  OutDataTypeStr=Inherit: Same as input  ParamDataTypeStr=Inherit: Same as input
  Integrator : Integrator
  Integrator1 : Integrator  InitialCondition=xpll0_pu
  Memory : Memory  InitialCondition=fb
  Selector : Selector  InputPortWidth=3  IndexOptions=Index vector (dialog)  Indices=2  OutputSizes=1
  Sqrt2 : Sqrt  SaturateOnIntegerOverflow=on
  Sum : Sum
  Sum1 : Sum  Inputs=++|
  Sum2 : Sum  Inputs=+++  InputSameDT=on  SaturateOnIntegerOverflow=on  OutDataTypeStr=Inherit: Same as first input
  abc to dq0 : powerlib_meascontrol/Transformations/abc to dq0  Alignment=90 degrees behind phase A axis
      settings: SourceProductBaseCode=MT,PS
  d²2 : Product  InputSameDT=on  RndMeth=Zero  SaturateOnIntegerOverflow=on  OutDataTypeStr=Inherit: Same as first input
  q²4 : Product  InputSameDT=on  RndMeth=Zero  SaturateOnIntegerOverflow=on  OutDataTypeStr=Inherit: Same as first input
  q²5 : Product  InputSameDT=on  RndMeth=Zero  SaturateOnIntegerOverflow=on  OutDataTypeStr=Inherit: Same as first input
  Freq : Outport  VectorParamsAs1DForOutWhenUnconnected=off
  wt : Outport  Port=2  VectorParamsAs1DForOutWhenUnconnected=off
  wires:
  Vabc/1 -> abc to dq0/1
  Integrator/1 -> wt/1, abc to dq0/2
  Memory/1 -> Freq/1
  Gain/1 -> Sum/1
  Gain1/1 -> Sum/2
  Integrator1/1 -> Gain1/1
  Demux2/1 -> d²2/1, d²2/2  "d"
  d²2/1 -> Sum2/1
  Demux2/3 -> q²5/1, q²5/2  "0"
  Demux2/2 -> q²4/1, q²4/2  "q"
  Sqrt2/1 -> Divide/1
  Sum2/1 -> Sqrt2/1
  q²5/1 -> Sum2/3
  abc to dq0/1 -> Demux2/1, Selector/1
  q²4/1 -> Sum2/2
  Selector/1 -> Divide/2  "Vq"
  Divide/1 -> Integrator1/1, Gain/1
  Gain10/1 -> First-Order Filter/1
  First-Order Filter/1 -> Memory/1
  Constant/1 -> Sum1/1
  Sum/1 -> Sum1/2  "W"
  Sum1/1 -> Integrator/1, Gain10/1  "W"

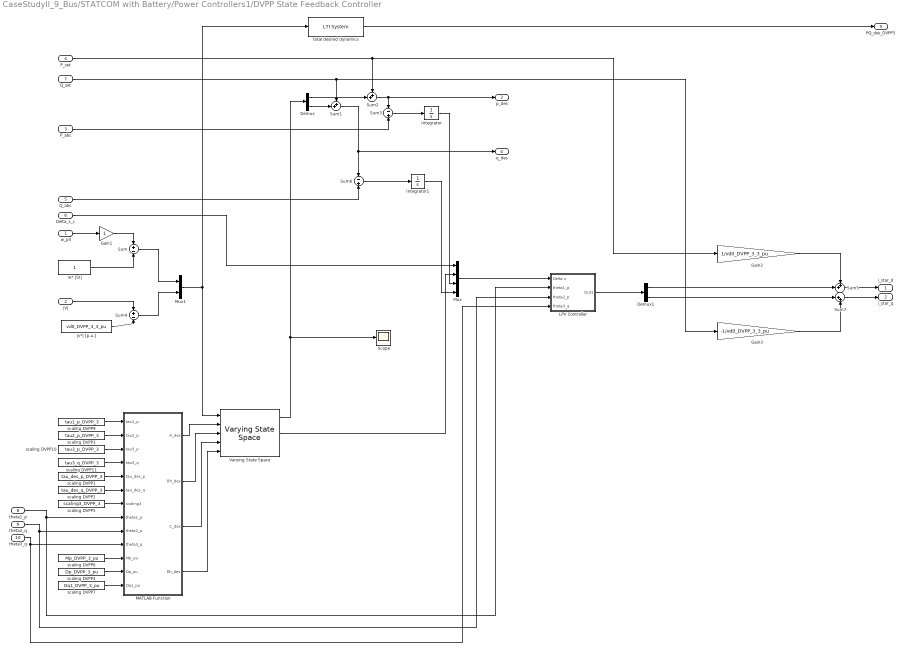
== system CaseStudyII_9_Bus/STATCOM with Battery/Power Controllers1/DVPP State Feedback Controller ==
  w_pll : Inport
  "|V| " : Inport  Port=2
  P_abc : Inport  Port=3
  P_set : Inport  Port=4
  Q_abc : Inport  Port=5
  Delta_x_c : Inport  Port=6
  Q_set : Inport  Port=7
  theta1_p : Inport  Port=8
  theta2_q : Inport  Port=9
  theta3_q : Inport  Port=10
  Demux : Demux  Outputs=2
  Demux1 : Demux  Outputs=2
  Gain1 : Gain
  Gain2 : Gain  Gain=1/vd0_DVPP_3_3_pu
  Gain3 : Gain  Gain=-1/vd0_DVPP_3_3_pu
  Integrator : Integrator
  Integrator1 : Integrator
  LPV Controller : Subsystem
  MATLAB Function : MATLAB Function  TreatAsAtomicUnit=on
  Mux : Mux
  Mux1 : Mux  Inputs=2
  Scope : Scope
  Sum : Sum  Inputs=+-
  Sum1 : Sum  Inputs=++|
  Sum2 : Sum  Inputs=++|
  Sum3 : Sum  Inputs=-+
  Sum4 : Sum  Inputs=+-
  Sum5 : Sum  Inputs=++|
  Sum6 : Sum  Inputs=-+
  Sum7 : Sum  Inputs=|++
  Varying State Space : cstblocks/Linear Parameter Varying/Varying State Space  x0=0  xNames=''  OutputX=on  OutputDX=on
  scaling DVPP1 : Constant  Value=tau_des_p_DVPP_3
  scaling DVPP10 : Constant  Value=tau3_p_DVPP_3
  scaling DVPP11 : Constant  Value=tau3_q_DVPP_3
  scaling DVPP2 : Constant  Value=tau_des_q_DVPP_3
  scaling DVPP3 : Constant  Value=tau2_p_DVPP_3
  scaling DVPP4 : Constant  Value=Dp_DVPP_3_pu
  scaling DVPP5 : Constant  Value=scaling3_DVPP_3
  scaling DVPP6 : Constant  Value=Mp_DVPP_3_pu
  scaling DVPP7 : Constant  Value=Dq1_DVPP_3_pu
  scaling DVPP9 : Constant  Value=tau1_p_DVPP_3
  total desired dynamics : cstblocks/LTI System  sys=T_des_DVPP_3  IC=pset
  w* [SI] : Constant
  |v*| [p.u.] : Constant  Value=vd0_DVPP_3_3_pu
  i_star_d : Outport
  i_star_q : Outport  Port=2
  p_des : Outport  Port=3
  q_des : Outport  Port=4
  PQ_des_DVPP3 : Outport  Port=5
  wires:
  Mux/1 -> LPV Controller/1(Delta x)
  Sum3/1 -> Integrator/1
  "|V| "/1 -> Sum4/1
  |v*| [p.u.]/1 -> Sum4/2
  w_pll/1 -> Gain1/1
  w* [SI]/1 -> Sum/2
  Sum/1 -> Mux1/1
  Mux1/1 -> total desired dynamics/1, Varying State Space/1
  Varying State Space/1 -> Demux/1, Scope/1
  P_abc/1 -> Sum3/2
  Q_abc/1 -> Sum6/2
  Sum6/1 -> Integrator1/1
  Integrator/1 -> Mux/3
  Integrator1/1 -> Mux/4
  Varying State Space/2 -> Mux/2
  Delta_x_c/1 -> Mux/1
  LPV Controller/1(Out1) -> Demux1/1
  Demux1/1 -> Sum5/2
  Gain1/1 -> Sum/1
  Sum4/1 -> Mux1/2
  Sum1/1 -> Sum6/1, q_des/1
  Demux/2 -> Sum1/2
  Q_set/1 -> Gain3/1, Sum1/1
  Demux/1 -> Sum2/2
  P_set/1 -> Gain2/1, Sum2/1
  Sum2/1 -> p_des/1, Sum3/1
  Sum5/1 -> i_star_d/1
  Gain2/1 -> Sum5/1
  Sum7/1 -> i_star_q/1
  Demux1/2 -> Sum7/1
  Gain3/1 -> Sum7/2
  scaling DVPP3/1 -> MATLAB Function/2(tau2_p)
  scaling DVPP10/1 -> MATLAB Function/3(tau3_p)
  scaling DVPP9/1 -> MATLAB Function/1(tau1_p)
  MATLAB Function/1(A_des) -> Varying State Space/2
  MATLAB Function/2(Bh_des) -> Varying State Space/3
  MATLAB Function/3(C_des) -> Varying State Space/4
  MATLAB Function/4(Dh_des) -> Varying State Space/5
  scaling DVPP6/1 -> MATLAB Function/11(Mp_pu)
  scaling DVPP4/1 -> MATLAB Function/12(Dp_pu)
  scaling DVPP7/1 -> MATLAB Function/13(Dq1_pu)
  theta2_q/1 -> LPV Controller/3(theta2_p), MATLAB Function/9(theta2_p)
  theta1_p/1 -> LPV Controller/2(theta1_p), MATLAB Function/8(theta1_p)
  theta3_q/1 -> MATLAB Function/10(theta3_q), LPV Controller/4(theta3_q)
  scaling DVPP5/1 -> MATLAB Function/7(scaling3)
  scaling DVPP2/1 -> MATLAB Function/6(tau_des_q)
  scaling DVPP1/1 -> MATLAB Function/5(tau_des_p)
  scaling DVPP11/1 -> MATLAB Function/4(tau3_q)
  total desired dynamics/1 -> PQ_des_DVPP3/1

== system CaseStudyII_9_Bus/Supercapacitor/PLL/Subsystem ==
  Vabc : Inport  PortDimensions=3
  Constant : Constant  Value=2*pi*50
  Demux2 : Demux  Outputs=3
  Divide : Product  Inputs=/*
  First-Order Filter : powerlib_meascontrol/Filters/First-Order Filter  FilterType=Lowpass  Tc=0.081  Ts=0  Initialize=on  Vac_Init=[0, 0, fb]  Vdc_Init=0  PlotResponse=off  FreqRange="[0,  200,  1]"
  Gain : Gain  Gain=kp_pll
  Gain1 : Gain  Gain=ki_pll
  Gain10 : Gain  Gain=1/2/pi  SaturateOnIntegerOverflow=on  OutDataTypeStr=Inherit: Same as input  ParamDataTypeStr=Inherit: Same as input
  Integrator : Integrator
  Integrator1 : Integrator  InitialCondition=xpll0_pu
  Memory : Memory  InitialCondition=fb
  Selector : Selector  InputPortWidth=3  IndexOptions=Index vector (dialog)  Indices=2  OutputSizes=1
  Sqrt2 : Sqrt  SaturateOnIntegerOverflow=on
  Sum : Sum
  Sum1 : Sum  Inputs=++|
  Sum2 : Sum  Inputs=+++  InputSameDT=on  SaturateOnIntegerOverflow=on  OutDataTypeStr=Inherit: Same as first input
  abc to dq0 : powerlib_meascontrol/Transformations/abc to dq0  Alignment=90 degrees behind phase A axis
      settings: SourceProductBaseCode=MT,PS
  d²2 : Product  InputSameDT=on  RndMeth=Zero  SaturateOnIntegerOverflow=on  OutDataTypeStr=Inherit: Same as first input
  q²4 : Product  InputSameDT=on  RndMeth=Zero  SaturateOnIntegerOverflow=on  OutDataTypeStr=Inherit: Same as first input
  q²5 : Product  InputSameDT=on  RndMeth=Zero  SaturateOnIntegerOverflow=on  OutDataTypeStr=Inherit: Same as first input
  Freq : Outport  VectorParamsAs1DForOutWhenUnconnected=off
  wt : Outport  Port=2  VectorParamsAs1DForOutWhenUnconnected=off
  wires:
  Vabc/1 -> abc to dq0/1
  Integrator/1 -> wt/1, abc to dq0/2
  Memory/1 -> Freq/1
  Gain/1 -> Sum/1
  Gain1/1 -> Sum/2
  Integrator1/1 -> Gain1/1
  Demux2/1 -> d²2/1, d²2/2  "d"
  d²2/1 -> Sum2/1
  Demux2/3 -> q²5/1, q²5/2  "0"
  Demux2/2 -> q²4/1, q²4/2  "q"
  Sqrt2/1 -> Divide/1
  Sum2/1 -> Sqrt2/1
  q²5/1 -> Sum2/3
  abc to dq0/1 -> Demux2/1, Selector/1
  q²4/1 -> Sum2/2
  Selector/1 -> Divide/2  "Vq"
  Divide/1 -> Integrator1/1, Gain/1
  Gain10/1 -> First-Order Filter/1
  First-Order Filter/1 -> Memory/1
  Constant/1 -> Sum1/1
  Sum/1 -> Sum1/2  "W"
  Sum1/1 -> Integrator/1, Gain10/1  "W"

== system CaseStudyII_9_Bus/Supercapacitor/Power Controllers/DVPP State Feedback Controller for Active Power Control ==
  w_pll : Inport
  P_abc : Inport  Port=2
  Delta_x_c : Inport  Port=3
  P_set : Inport  Port=4
  Constant : Constant  Value=ReferenceSS3_DVPP_1.A  VectorParams1D=off
  Constant1 : Constant  Value=ReferenceSS3_DVPP_1.B  VectorParams1D=off
  Constant2 : Constant  Value=ReferenceSS3_DVPP_1.C  VectorParams1D=off
  Constant3 : Constant  Value=ReferenceSS3_DVPP_1.D  VectorParams1D=off
  Gain : Gain  Gain=K3_DVPP_1  Multiplication=Matrix(K*u)
  Gain1 : Gain
  Gain2 : Gain  Gain=1/vd0_DVPP_1_3_pu
  Integrator : Integrator
  Mux : Mux  Inputs=3
  Scope : Scope
  Sum : Sum  Inputs=+-
  Sum1 : Sum  Inputs=++|
  Sum2 : Sum  Inputs=++|
  Sum3 : Sum  Inputs=-+
  Varying State Space : cstblocks/Linear Parameter Varying/Varying State Space  x0=0  xNames=''  OutputX=on  OutputDX=on
  w* [SI] : Constant
  p_des : Outport
  i_star_d : Outport  Port=2
  wires:
  Mux/1 -> Gain/1
  Varying State Space/1 -> Sum1/2, Scope/1
  Sum3/1 -> Integrator/1
  w_pll/1 -> Gain1/1
  w* [SI]/1 -> Sum/2
  P_abc/1 -> Sum3/2
  Integrator/1 -> Mux/3
  Varying State Space/2 -> Mux/2
  Delta_x_c/1 -> Mux/1
  Gain/1 -> Sum2/1
  Gain1/1 -> Sum/1
  Constant/1 -> Varying State Space/2
  Constant1/1 -> Varying State Space/3
  Constant2/1 -> Varying State Space/4
  Constant3/1 -> Varying State Space/5
  Sum/1 -> Varying State Space/1
  Sum1/1 -> Sum3/1, p_des/1
  P_set/1 -> Gain2/1, Sum1/1
  Gain2/1 -> Sum2/2
  Sum2/1 -> i_star_d/1
